simulink model "dynamics_mean"  (R2023a)
settings: Solver=ode4  StartTime=0.0  StopTime=t_duration  FixedStep=dt  MaxStep=max_step_size  RelTol=relative_tolerance
undefined symbols (not defined in the file): chief, deputy1, deputy2, environment
settings Model: Creator=ndelurgio  LastModifiedBy=ndelurgio

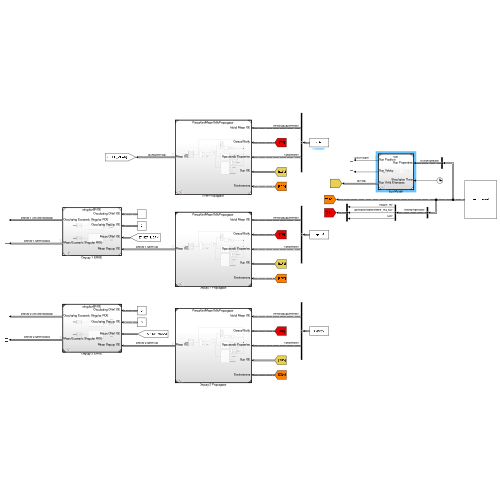
[thumbnail: Simulink's stored preview of the top-level diagram]
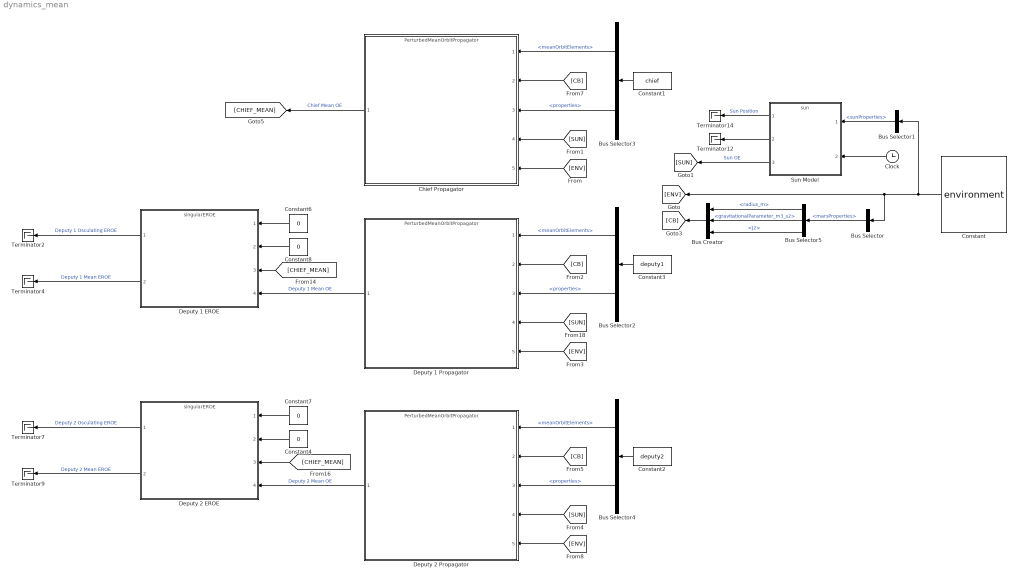
== system dynamics_mean ==
  Bus Creator : BusCreator  Inputs=3  OutDataTypeStr=Bus: planetProperties  NonVirtualBus=on
      settings: InheritFromInputs=off
  Bus Selector : BusSelector  OutputSignals=marsProperties
  Bus Selector1 : BusSelector  OutputSignals=sunProperties
  Bus Selector2 : BusSelector  OutputSignals=initialConditions.meanOrbitElements,properties
  Bus Selector3 : BusSelector  OutputSignals=initialConditions.meanOrbitElements,properties
  Bus Selector4 : BusSelector  OutputSignals=initialConditions.meanOrbitElements,properties
  Bus Selector5 : BusSelector  OutputSignals=radius_m,gravitationalParameter_m3_s2,J2
  Chief Propagator : ModelReference  ModelNameDialog=PerturbedMeanOrbitPropagator  SimulationMode=Normal  ModelReferenceVersion=1.207
  Clock : Clock
  Constant : Constant  Value=environment  OutDataTypeStr=Bus: environmentBus
  Constant1 : Constant  Value=chief  OutDataTypeStr=Bus: chiefBus
  Constant2 : Constant  Value=deputy2  OutDataTypeStr=Bus: deputy1Bus
  Constant3 : Constant  Value=deputy1  OutDataTypeStr=Bus: deputy1Bus
  Constant{4,6..8} (4 alike) : Constant  Value=0  OutDataTypeStr=Bus: osculatingOrbitElements
  Deputy 1 EROE : ModelReference  ModelNameDialog=singularEROE  SimulationMode=Normal  ModelReferenceVersion=1.18
  Deputy 1 Propagator : ModelReference  ModelNameDialog=PerturbedMeanOrbitPropagator  SimulationMode=Normal  ModelReferenceVersion=1.207
  Deputy 2 EROE : ModelReference  ModelNameDialog=singularEROE  SimulationMode=Normal  ModelReferenceVersion=1.18
  Deputy 2 Propagator : ModelReference  ModelNameDialog=PerturbedMeanOrbitPropagator  SimulationMode=Normal  ModelReferenceVersion=1.207
  Sun Model : ModelReference  ModelNameDialog=sun  SimulationMode=Normal  ModelReferenceVersion=1.19
  Terminator{2,4,7,9,12,14} (6 alike) : Terminator
  wires:
  Constant/1 -> [ENV], Bus Selector/1, Bus Selector1/1
  [ENV] -> Chief Propagator/5
  Constant1/1 -> Bus Selector3/1
  Bus Selector1/1 -> Sun Model/1  "<sunProperties>"
  Clock/1 -> Sun Model/2
  Sun Model/1 -> Terminator14/1  "Sun Position"
  [SUN] -> Chief Propagator/4
  Chief Propagator/1 -> [CHIEF_MEAN]  "Chief Mean OE"
  Bus Selector3/2 -> Chief Propagator/3  "<properties>"
  Bus Selector3/1 -> Chief Propagator/1  "<meanOrbitElements>"
  Deputy 1 Propagator/1 -> Deputy 1 EROE/4  "Deputy 1 Mean OE"
  Bus Selector/1 -> Bus Selector5/1  "<marsProperties>"
  [CB] -> Chief Propagator/2
  Bus Selector2/1 -> Deputy 1 Propagator/1  "<meanOrbitElements>"
  Bus Selector2/2 -> Deputy 1 Propagator/3  "<properties>"
  Constant3/1 -> Bus Selector2/1
  [CHIEF_MEAN] -> Deputy 1 EROE/3
  Deputy 1 EROE/1 -> Terminator2/1  "Deputy 1 Osculating EROE"
  Deputy 1 EROE/2 -> Terminator4/1  "Deputy 1 Mean EROE"
  [CHIEF_MEAN] -> Deputy 2 EROE/3
  Constant7/1 -> Deputy 2 EROE/1
  Deputy 2 EROE/2 -> Terminator9/1  "Deputy 2 Mean EROE"
  Deputy 2 Propagator/1 -> Deputy 2 EROE/4  "Deputy 2 Mean OE"
  Deputy 2 EROE/1 -> Terminator7/1  "Deputy 2 Osculating EROE"
  Bus Creator/1 -> [CB]
  Bus Selector5/1 -> Bus Creator/1  "<radius_m>"
  Bus Selector5/2 -> Bus Creator/2  "<gravitationalParameter_m3_s2>"
  Bus Selector5/3 -> Bus Creator/3  "<J2>"
  Sun Model/2 -> Terminator12/1
  Sun Model/3 -> [SUN]  "Sun OE"
  [SUN] -> Deputy 1 Propagator/4
  [ENV] -> Deputy 1 Propagator/5
  [CB] -> Deputy 1 Propagator/2
  Constant2/1 -> Bus Selector4/1
  [ENV] -> Deputy 2 Propagator/5
  Bus Selector4/1 -> Deputy 2 Propagator/1  "<meanOrbitElements>"
  [SUN] -> Deputy 2 Propagator/4
  Bus Selector4/2 -> Deputy 2 Propagator/3  "<properties>"
  [CB] -> Deputy 2 Propagator/2
  Constant4/1 -> Deputy 2 EROE/2
  Constant8/1 -> Deputy 1 EROE/2
  Constant6/1 -> Deputy 1 EROE/1
